simulink model "HW"  (R2022b)
settings: Solver=VariableStepAuto  StartTime=0.0  StopTime=10.0  FixedStep=0.0001  MaxStep=0.001  RelTol=1e-3
values from neighbouring files (symbols this model uses):
  a_sin = [pi/2; pi/2; 0.2; pi/2]    [HW_par.m]
  Kd = 1000*eye(4)    [HW_par.m]
  Kp = 1000*eye(4)    [HW_par.m]
  omega_sin = 10*[1; 1; 1; 1]    [HW_par.m]
  q_0 = [pi/2;pi/4;0;0]    [HW_par.m]    (also in SCARA_inv_diff_kin.m = [-pi/4,pi/4,-0.15,0])
  q_dot_0 = [0;0;0;0]    [HW_par.m]
  q_target = [pi/2; pi/3; 0.1; -pi/4]    [HW_par.m]
undefined symbols (not defined in the file or in its folder): a_filt, b_filt
settings Model: Creator=Alberto  LastModifiedBy=Christian Russo
settings SolverCC: AlgebraicLoopSolver=TrustRegion
settings DebuggingCC: UnconnectedInputMsg=warning  UnconnectedOutputMsg=warning  UnconnectedLineMsg=warning  SFMachineParentedDataDiag=warning
settings ModelReferenceCC: EnableRefExpFcnMdlSchedulingChecks=on
settings RTWCC: DLArmComputeVersion=19.05

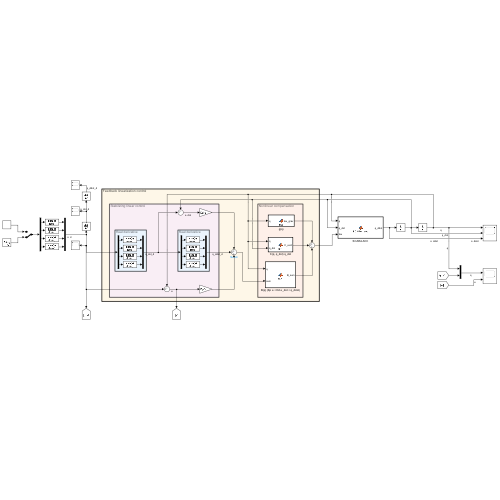
[thumbnail: Simulink's stored preview of the top-level diagram]
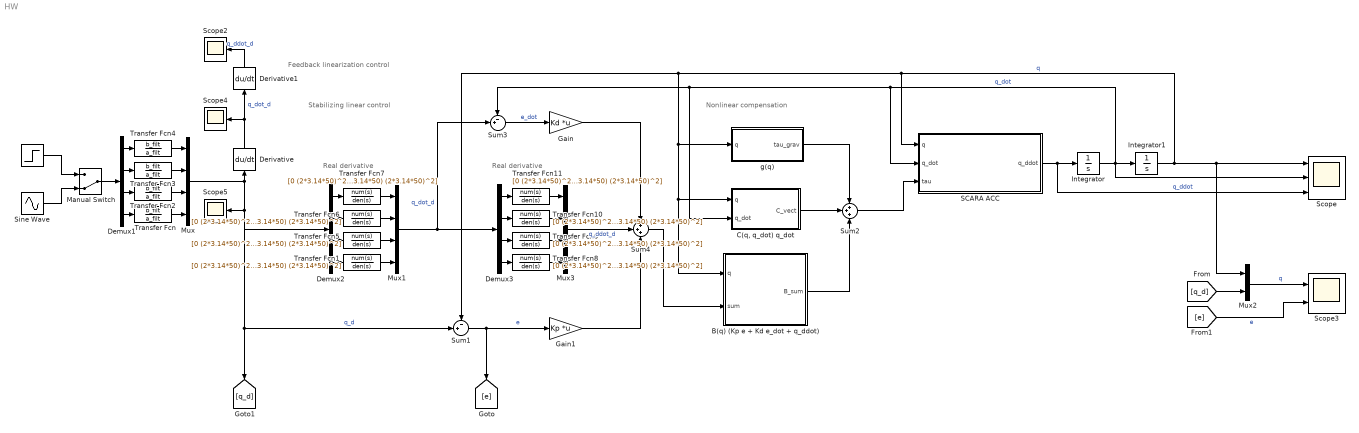
== system HW ==
  note: Feedback linearization control
  note: Real derivative
  note: Real derivative
  note: Stabilizing linear control
  note: Nonlinear compensation
  " " : Step  After=q_target  SampleTime=0
  B(q) (Kp e + Kd e_dot + q_ddot) : MATLAB Function  TreatAsAtomicUnit=on
  "C(q, q_dot) q_dot" : MATLAB Function  TreatAsAtomicUnit=on
  Demux1 : Demux
  Demux2 : Demux
  Demux3 : Demux
  Derivative : Derivative
  Derivative1 : Derivative
  Gain : Gain  Gain=Kd  Multiplication=Matrix(K*u)
  Gain1 : Gain  Gain=Kp  Multiplication=Matrix(K*u)
  Integrator : Integrator  InitialCondition=q_dot_0
  Integrator1 : Integrator  InitialCondition=q_0
  Manual Switch : ManualSwitch  CurrentSetting=0
  Mux : Mux
  Mux1 : Mux
  Mux2 : Mux  Inputs=2
  Mux3 : Mux
  SCARA ACC : MATLAB Function  TreatAsAtomicUnit=on
  Scope : Scope  NumInputPorts=3
  Scope2 : Scope
  Scope3 : Scope  NumInputPorts=2
  Scope4 : Scope
  Scope5 : Scope
  Sine Wave : Sin  Amplitude=a_sin  Frequency=omega_sin  SampleTime=0
  Sum1 : Sum  Inputs=-+|
  Sum2 : Sum  Inputs=+++
  Sum3 : Sum  Inputs=-+|
  Sum4 : Sum  Inputs=+++
  Transfer Fcn{,2..4} (4 alike) : TransferFcn  Numerator=b_filt  Denominator=a_filt
  Transfer Fcn{1,5..11} (8 alike) : TransferFcn  Numerator=[0 (2*3.14*50)^2 0]  Denominator=[1 2*(1/sqrt(2))*(2*3.14*50) (2*3.14*50)^2]
  g(q) : MATLAB Function  TreatAsAtomicUnit=on
  wires:
  SCARA ACC/1(q_ddot) -> Integrator/1, Scope/3  "q_ddot"
  Demux1/1 -> Transfer Fcn4/1
  Demux1/2 -> Transfer Fcn3/1
  Demux1/3 -> Transfer Fcn2/1
  Demux1/4 -> Transfer Fcn/1
  Transfer Fcn4/1 -> Mux/1
  Transfer Fcn3/1 -> Mux/2
  Transfer Fcn2/1 -> Mux/3
  Transfer Fcn/1 -> Mux/4
  Mux/1 -> [q_d], Sum1/2, Scope5/1, Demux2/1, Derivative/1  "q_d"
  " "/1 -> Manual Switch/1
  Sine Wave/1 -> Manual Switch/2
  Derivative/1 -> Derivative1/1, Scope4/1  "q_dot_d"
  Derivative1/1 -> Scope2/1  "q_ddot_d"
  Mux2/1 -> Scope3/1  "q"
  [q_d] -> Mux2/2
  Integrator/1 -> Sum3/1, "C(q, q_dot) q_dot"/2(q_dot), SCARA ACC/2(q_dot), Integrator1/1, Scope/2  "q_dot"
  [e] -> Scope3/2  "e"
  Integrator1/1 -> Sum1/1, g(q)/1(q), "C(q, q_dot) q_dot"/1(q), B(q) (Kp e + Kd e_dot + q_ddot)/1(q), SCARA ACC/1(q), Mux2/1, Scope/1  "q"
  Demux2/4 -> Transfer Fcn1/1
  Transfer Fcn7/1 -> Mux1/1
  Transfer Fcn1/1 -> Mux1/4
  Demux2/3 -> Transfer Fcn5/1
  Demux2/1 -> Transfer Fcn7/1
  Transfer Fcn5/1 -> Mux1/3
  Demux2/2 -> Transfer Fcn6/1
  Transfer Fcn6/1 -> Mux1/2
  Manual Switch/1 -> Demux1/1
  Transfer Fcn8/1 -> Mux3/4
  Demux3/2 -> Transfer Fcn10/1
  Transfer Fcn9/1 -> Mux3/3
  Demux3/3 -> Transfer Fcn9/1
  Demux3/4 -> Transfer Fcn8/1
  Demux3/1 -> Transfer Fcn11/1
  Transfer Fcn11/1 -> Mux3/1
  Transfer Fcn10/1 -> Mux3/2
  Mux1/1 -> Demux3/1, Sum3/2  "q_dot_d"
  Sum3/1 -> Gain/1  "e_dot"
  Sum2/1 -> SCARA ACC/3(tau)
  "C(q, q_dot) q_dot"/1(C_vect) -> Sum2/2
  g(q)/1(tau_grav) -> Sum2/1
  B(q) (Kp e + Kd e_dot + q_ddot)/1(B_sum) -> Sum2/3
  Sum4/1 -> B(q) (Kp e + Kd e_dot + q_ddot)/2(sum)
  Mux3/1 -> Sum4/2  "q_ddot_d"
  Gain/1 -> Sum4/1
  Gain1/1 -> Sum4/3
  Sum1/1 -> Gain1/1, [e]  "e"

== matlab function HW/g(q) ==
  data: q input; tau_grav output
function tau_grav = fcn(q)%#codegen
coder.extrinsic('f_g_vect_mex');
tau_grav = zeros(4,1);
tau_grav = reshape(full(f_g_vect_mex('f_g_vect', q)),4,1);

== matlab function HW/B(q) (Kp e + Kd e_dot + q_ddot) ==
  data: q input; B_sum output; sum input
function B_sum = fcn(q, sum)%#codegen
coder.extrinsic('f_B_mex'); 
B = eye(4);
B = full(f_B_mex('f_B',q));
B_sum = B * sum;

== matlab function HW/C(q, q_dot) q_dot ==
  data: q input; q_dot input; C_vect output
function C_vect = fcn(q, q_dot)%#codegen
coder.extrinsic('f_C_vect_mex'); 
C_vect = zeros(4,1);
C_vect = reshape(full(f_C_vect_mex('f_C_vect', q, q_dot)),4 ,1);

== matlab function HW/SCARA ACC ==
  data: q input; q_ddot output; q_dot input; tau input
function q_ddot = SCARA_acc(q, q_dot, tau)%#codegen
coder.extrinsic('f_B_mex'); 
coder.extrinsic('f_C_vect_mex'); 
coder.extrinsic('f_g_vect_mex');
B = eye(4);
C_vect = zeros(4,1);
F_g = zeros(4,1);
tau = reshape(tau,4,1);
q_ddot = zeros(4,1);
B = full(f_B_mex('f_B',q));
C_vect = full(f_C_vect_mex('f_C_vect', q, q_dot));
F_g = full(f_g_vect_mex('f_g_vect', q));
q_ddot = (eye(4)/B)*(-C_vect-F_g+tau);
